simulink model "Aircraft_Flight_Dynamic_Model"  (R2015b)
settings: Solver=ode45  StartTime=0.0  StopTime=120  RelTol=1e-3
InitFcn:
  | Aircraft_Longitudinal_Matrix
  | Pre_3D_Visualisation
values from neighbouring files (symbols this model uses):
  A_AC = [Xu_Mean,                 Xw,             0,                     -g;      Zu_Mean,                    Zw,               u0_Mean,              0;      Mu + (Mw_dot*Zu_Mean), Mw + (Mw_dot*Zw), Mq + (Mw_dot*u0_Mean*26.5),       0;      0,                     0,                1,                         0]    [Aircraft_Longitudinal_Matrix.m]
  A_Lat = [Yv,               Yp,               -(u0_Mean - Yr),              -g*cos(theta0);         Lv,               Lp,                            Lr,               0;       Nv,               Np,                            Nr,               0;      0,                 1,                             0,               0]    [Aircraft_Lateral_Matrix.m]    (also in eurostar.mat = [-0.00450002280245 -0.270072142257 0.00607503078331 0 0 -10.)
  B_AC = [0               Xdt;         Z_deltae            0;          M_deltae+Mw_dot*Z_deltae     M_deltat+Mw_dot*Z_deltat;         0            0]    [Aircraft_Longitudinal_Matrix.m]
  B_Lat = [0          (Ydr/u0_Mean);         Lda                  Ldr;         Nda                  Ndr;         0                      0]    [Aircraft_Lateral_Matrix.m]    (also in eurostar.mat = [0  0.0721546662292; -9.05833694873  -7.89708361128e-05; 8.8)
  C_AC = eye(4)    [Aircraft_Longitudinal_Matrix.m]
  C_Lat = eye(4)    [Aircraft_Lateral_Matrix.m]    (also in eurostar.mat = [1 0 0 0 0 1 0 0 0 0 1 0 ... (16 elements, 4x4)])
  D_AC = zeros(4,2)    [Aircraft_Longitudinal_Matrix.m]
  D_Lat = zeros(4,2)    [Aircraft_Lateral_Matrix.m]    (also in eurostar.mat = [0  0; 0  0; 0  0; 0  0])
  initial = [0; 0; 0; 0; 0; 0; 0; 0]    [Aircraft_Lateral_Matrix.m]    (also in Aircraft_Longitudinal_Matrix.m = [u0_Mean; 0; 0; 0; 0; 0; 0; 0]; eurostar.mat = [0 0 0 0 0 0 0 0])
  V = V./(scale_factor*correction)    [Pre_3D_Visualisation.m]
  x0 = [10 0 0 10*(pi/180)]    [Aircraft_Longitudinal_Matrix.m]
  x_Lat = [0 0 0 0]    [Aircraft_Lateral_Matrix.m]    (also in eurostar.mat)
undefined symbols (not defined in the file or in its folder): F
libraries: simulink x4, realtime_pacer_lib x1
settings Model: Creator=p-narayan  LastModifiedBy=Joseph
settings DataIOCC: SaveFormat=Array
settings DebuggingCC: SolverPrmCheckMsg=warning
settings HardwareCC: ProdBitPerPointer=32  ProdLargestAtomicFloat=None  ProdIntDivRoundTo=Undefined  ProdEndianess=Unspecified  ProdWordSize=32  ProdHWDeviceType=32-bit Generic
settings GRTTargetCC: GeneratePreprocessorConditionals=Disable all
settings ConfigComp: CovModelRefEnable=Off  CovSFcnEnable=off

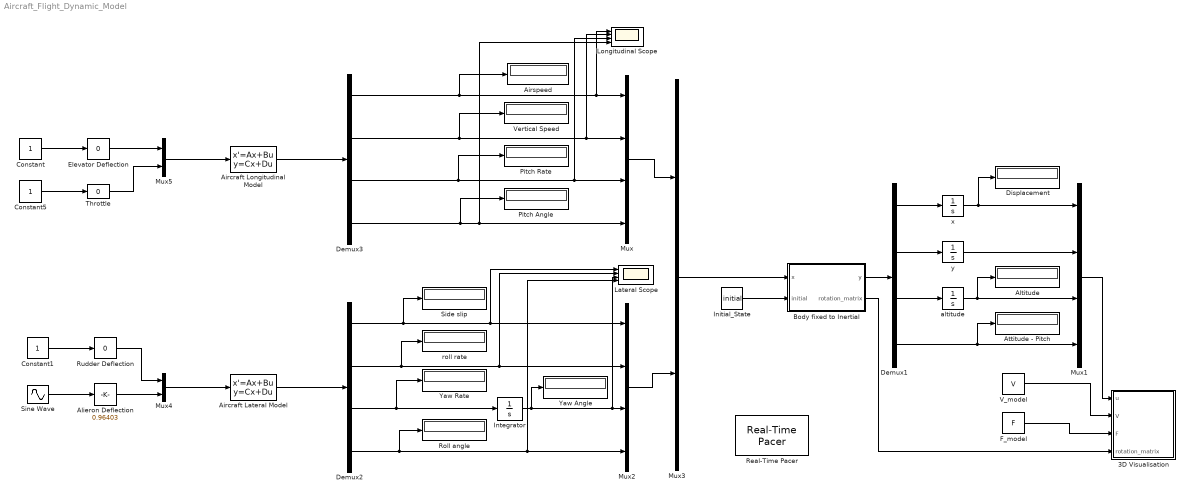
== system Aircraft_Flight_Dynamic_Model ==
  3D Visualisation : MATLAB Function  TreatAsAtomicUnit=on
  Aircraft Lateral Model : StateSpace  A=A_Lat  B=B_Lat  C=C_Lat  D=D_Lat  X0=x_Lat
  Aircraft Longitudinal Model : StateSpace  A=A_AC  B=B_AC  C=C_AC  D=D_AC  X0=x0
  Airspeed : Display
  Alieron Deflection : simulink/Math Operations/Slider Gain  low=0  gain=0.96403  high=2
  Altitude : Display
  Attitude - Pitch : Display
  Body fixed to Inertial : MATLAB Function  TreatAsAtomicUnit=on
  Constant : Constant
  Constant1 : Constant  SampleTime=0.1
  Constant5 : Constant
  Demux1 : Demux
  Demux2 : Demux
  Demux3 : Demux
  Displacement : Display
  Elevator Deflection : simulink/Math Operations/Slider Gain  low=0  gain=0  high=2
  F_model : Constant  Value=F
  Initial_State : Constant  Value=initial  SampleTime=0.1
  Integrator : Integrator
  Lateral Scope : Scope  NumInputPorts=4
  Longitudinal Scope : Scope  NumInputPorts=4
  Mux : Mux
  Mux1 : Mux
  Mux2 : Mux
  Mux3 : Mux  Inputs=2
  Mux4 : Mux  Inputs=2
  Mux5 : Mux  Inputs=2
  Pitch Angle : Display
  Pitch Rate : Display
  Real-Time Pacer : realtime_pacer_lib/Real-Time Pacer  simTimePerRealTime=10
  Roll angle : Display
  Rudder Deflection : simulink/Math Operations/Slider Gain  low=0  gain=0  high=2
  Side slip : Display
  Sine Wave : Sin  Amplitude=0.1  SampleTime=0
  "Throttle " : simulink/Math Operations/Slider Gain  low=0  gain=0  high=2
  "V_model " : Constant  Value=V
  Vertical Speed : Display
  Yaw Angle : Display
  Yaw Rate : Display
  altitude : Integrator  InitialCondition=500  ContinuousStateAttributes='altitude'
  roll rate : Display
  x : Integrator
  y : Integrator
  wires:
  Body fixed to Inertial/1(y) -> Demux1/1
  Demux1/1 -> x/1
  Demux1/2 -> y/1
  Demux1/3 -> altitude/1
  Demux1/4 -> Mux1/4, Attitude - Pitch/1
  altitude/1 -> Mux1/3, Altitude/1
  y/1 -> Mux1/2
  Mux1/1 -> 3D Visualisation/1(u)
  "V_model "/1 -> 3D Visualisation/2(V)
  F_model/1 -> 3D Visualisation/3(F)
  Initial_State/1 -> Body fixed to Inertial/2(initial)
  x/1 -> Displacement/1, Mux1/1
  Body fixed to Inertial/2(rotation_matrix) -> 3D Visualisation/4(rotation_matrix)
  Aircraft Lateral Model/1 -> Demux2/1
  Aircraft Longitudinal Model/1 -> Demux3/1
  Mux3/1 -> Body fixed to Inertial/1(x)
  Mux/1 -> Mux3/1
  Mux2/1 -> Mux3/2
  Demux2/3 -> Integrator/1, Yaw Rate/1
  Demux2/4 -> Roll angle/1, Mux2/4, Lateral Scope/4
  Demux2/2 -> Lateral Scope/2, Mux2/2, roll rate/1
  Demux2/1 -> Mux2/1, Lateral Scope/1, Side slip/1
  Demux3/2 -> Longitudinal Scope/2, Mux/2, Vertical Speed/1
  Demux3/3 -> Longitudinal Scope/3, Mux/3, Pitch Rate/1
  Demux3/4 -> Pitch Angle/1, Mux/4, Longitudinal Scope/4
  Integrator/1 -> Yaw Angle/1, Lateral Scope/3, Mux2/3
  Mux4/1 -> Aircraft Lateral Model/1
  Mux5/1 -> Aircraft Longitudinal Model/1
  Elevator Deflection/1 -> Mux5/1
  "Throttle "/1 -> Mux5/2
  Constant/1 -> Elevator Deflection/1
  Constant5/1 -> "Throttle "/1
  Constant1/1 -> Rudder Deflection/1
  Rudder Deflection/1 -> Mux4/1
  Alieron Deflection/1 -> Mux4/2
  Sine Wave/1 -> Alieron Deflection/1
  Demux3/1 -> Longitudinal Scope/1, Mux/1, Airspeed/1

== matlab function Aircraft_Flight_Dynamic_Model/3D Visualisation ==
  data: u input; V input; F input; rotation_matrix input
function fcn(u, V, F, rotation_matrix)
%#codegen

% opengl hardware
coder.extrinsic('patch')
coder.extrinsic('delete')
coder.extrinsic('exist')

cla

% Frame = struct('cdata',zeros(420,560,3));

%
x = u(1);
y = u(2);
z = u(3);
% pitch = u(4);

% % x = u(1);
% % y = 0;
% % z = u(3);
% % pitch = u(4);
% % roll = 0;
% % yaw = 0;
% % scale_factor = 1;
% % step = 0.1;
% % % selector

% coder.extrinsic('set_param');
% coder.extrinsic('trajectory3');
% coder.extrinsic('delete');

% =========================================================================

% trajectory3(x,0,z,pitch,0,0,0.2,0.1,'helicopter')

% trajectory3(x,y,z,pitch,roll,yaw,scale_factor,step,selector,varargin);

% mov=nargout;

%  strcmp(selector,'helicopter')
%     load helicopter;
% % V_AC=[-V(:,2) V(:,1) V(:,3)];
% % V_AC(:,1)=V_AC(:,1)-round(sum(V_AC(:,1))/size(V_AC,1));
% % V_AC(:,2)=V_AC(:,2)-round(sum(V_AC(:,2))/size(V_AC,1));
% % V_AC(:,3)=V_AC(:,3)-round(sum(V_AC(:,3))/size(V_AC,1));
% % 
% % correction=max(abs(V_AC(:,1)));
% % V_AC=V_AC./(scale_factor*correction);
% ii=length(x);
% resto=mod(ii,step);

%%%%%%%%%%%%%%%needed for the transformation%%%%%%%%%%%%%%%

% y=y;
% z=z;
% pitch=pitch;
% roll=roll;
% yaw=-yaw;

%%%%%%%%%%%%%%%%%%%%%%%%%%%%%%%%%%%%%%%%%%%%%%%%%%%%%%%%%%%%

% % frame = 0;
% for i=1:step:(ii-resto)
%     if mov | (i == 1)
%         clf;
%         plot3(x,y,z);
%         grid on;
%         hold on;
%         light;
%     end

% theta=pitch;
% phi=-roll;
% psi=yaw;

%%%%%%%%%%%%%%%%%%%%%%%%%%%%%%%%%%%%%%%%%%%%%%%%%%%%%%%%%%%%%%

% Tbe=[cos(psi)*cos(theta), -sin(psi)*cos(theta), sin(theta);
%     cos(psi)*sin(theta)*sin(phi)+sin(psi)*cos(phi) ...
%     -sin(psi)*sin(theta)*sin(phi)+cos(psi)*cos(phi) ...
%     -cos(theta)*sin(phi);
%     -cos(psi)*sin(theta)*cos(phi)+sin(psi)*sin(phi) ...
%     sin(psi)*sin(theta)*cos(phi)+cos(psi)*sin(phi) ...
%     cos(theta)*cos(phi)];

%%%%%%%%%%%%%%%%%%%%%%%%%%%%%%%%%%%%%%%%%%%%%%%%%%%%%%%%%%%%%%

% Vnew=V*Tbe;
Vnew=V*rotation_matrix;
rif=[x y z];
X0=repmat(rif,size(Vnew,1),1);
Vnew=Vnew+X0;

p = patch('faces', F, 'vertices' ,Vnew);
set(p, 'facec', [1 0 0]);
set(p, 'EdgeColor','none');

% output = getframe(1);
% outputfile =  
% imwrite(img, 'outputfile.jpg');
% Frame = [1 1];





% if mov | (i == 1)
%     view(theView);
%     axis equal;
% end

% if mov
%     if i == 1
%         ax = axis;
%     else
%         axis(ax);
%     end
%     lighting phong
%     frame = frame + 1;
%     M(frame) = getframe;
% end

% end

% hold on;
% plot3(x,y,z);

% view(theView);
% daspect([1 1 1]) ;
% xlabel('X');
% ylabel('Y');
% zlabel('Z');

% cd (cur_dir);

% =========================================================================

== matlab function Aircraft_Flight_Dynamic_Model/Body fixed to Inertial ==
  data: x input; y output; initial input; rotation_matrix output
function [y, rotation_matrix] = fcn(x, initial)
%#codegen

% xdot = Ax + Bu
% where x = [Delta_u, Delta_w, Delta_q, Delta_theta]
% and y = [x_dot, y_dot, z_dot, Delta_theta]     % aircraft speed in
% inertial axis and pitch angle

theta = x(4)+initial(4);
psi = x(7)+initial(7);
phi = x(8)+initial(8);
    
u_b = x(1)+initial(1);
v_b = x(5)+initial(5);
w_b = x(2)+initial(2);

uvw_b = [u_b; v_b; w_b];

r11 = cos(theta)*cos(psi);
r12 = (sin(phi)*sin(theta)*cos(psi))-(cos(phi)*sin(psi));
r13 = (sin(phi)*sin(psi))+(cos(phi)*sin(theta)*cos(psi));

r21 = cos(theta)*sin(psi);
r22 = (cos(phi)*cos(psi))+sin(phi)*sin(theta)*sin(psi);
r23 = (cos(phi)*sin(theta)*sin(psi))-(sin(phi)*cos(psi));

r31 = -sin(theta);
r32 = sin(phi)*cos(theta);
r33 = cos(phi)*cos(theta);

rotation_matrix = [r11, r12, r13;...
                   r21, r22, r23;...
                   r31, r32, r33];

v_i = rotation_matrix*uvw_b;

y = [v_i(1), v_i(2), v_i(3), theta];
